simulink library "RxTxFixedPointLibrary"  (R2018a)
settings: Solver=VariableStepAuto  StartTime=0.0  StopTime=10.0  RelTol=1e-3
values from neighbouring files (symbols this model uses):
  AGCBarkerSymbols = 160 + 28    (= 188)    [modelSettings.m]
  coeff = rcosdesign(beta, span, sps, 'sqrt') * filterGain    [modelSettings.m]
  crcDecodeLag = length(crc32Poly) - 1 + 2    [modelSettings.m]
  CRCGeneratorLag = 34    [modelSettings.m]
  EQTrainingSymbols = 250    [modelSettings.m]
  K1 = fi(K1, 0)    [modelSettings.m]
  K2 = fi(K2, 0)    [modelSettings.m]
  numHeaderBits = 16    [modelSettings.m]
  numTrainingSamples = 250    [modelSettings.m]
  pLen = uint16(length(PreambleBarkersBits))    [modelSettings.m]
  RadioSampleRate = 1e6    (= 1000000)    [modelSettings.m]
  samplesPerSymbol = 4    [modelSettings.m]
  VibertiTracebackLength = 34 + 0    (= 34)    [modelSettings.m]
  xPreambleSeq = hPSKModTrain(seq)    [modelSettings.m]
undefined symbols (not defined in the file or in its folder): j
libraries: simulink x25, dsphdlfiltering x20, hdlsllib x10, commseqgen3 x4, commdigbbndpm3 x3, commcrc2 x2, commcnvcod2 x2, dspsigops x2, dspstat3 x1, commfilt2 x1
(part 3 of 3)

== matlab function RxTxFixedPointLibrary/Receiver_HDL/Viterbi Decode/Buffer/DEBUG: Vitberi Check/MATLAB Function2 ==
  data: bits input; enable input; reset input; crc input
function fcn(bits, enable, reset, crc)
 
persistent buffer index crcEnc crcDec txData

trellis = poly2trellis(7,[171 133]);
tbl = 34;

if isempty(buffer)
    buffer = false(4000,1);
    index = uint16(1);
    ply = 'z^32 + z^26 + z^23 + z^22 + z^16 + z^12 + z^11 + z^10 + z^8 + z^7 + z^5 + z^4 + z^2 + z + 1';
    crcEnc = comm.CRCGenerator('Polynomial',ply);
    crcDec = comm.CRCDetector ('Polynomial',ply);
    rate = 1/2;
    txData = repmat(logical([0;1]), 8*200*log2(4)*rate/2, 1); % Repeating [0 1]
end

if enable
    if reset
       index = uint16(1); 
    end
    
    buffer(index:index+1) = bits;
    index = index + uint16(2);
    if crc%index>3480
        % Generate true data
        crctx = crcEnc(txData);
        dataHardtx = convenc(crctx,trellis);
        % Check
        crcrx = vitdec(buffer(1:3264+tbl*2),trellis,tbl,'cont','hard');
        [rxData,e2] = crcDec(crcrx(tbl+1:tbl+1632));
        % Double check
        crcrx2 = vitdec([dataHardtx;false(tbl*2,1)],trellis,tbl,'cont','hard');
        [rxData2,e2] = crcDec(crcrx2(tbl+1:tbl+1632));
        %[dataHardtx buffer(1:3264)]
        disp(e2);
    end
    if index>4000
        index = uint16(1);
    end
end

== matlab function RxTxFixedPointLibrary/Transmitter_HDL/Packet Generation/Payload/MATLAB Function ==
  data: enable input; reset output; mode output
function [reset,mode] = fcn(enable)

persistent counter

if isempty(counter)
   counter = uint8(0);
end

if enable
    counter = uint8(34*2); % tracebacklength*2
    mode = uint8(1);
    reset = true;
elseif counter>uint8(0)
    counter = counter - 1;
    mode = uint8(1);
    reset = false;
else
    mode = uint8(0);
    reset = false;
end

== matlab function RxTxFixedPointLibrary/Receiver_HDL/Frame Recover/Gardner Timing Recovery/TED Lock Detector/MATLAB Function ==
  data: u input; y output
function y = abs(u)

y = fi(u,0,16,15);

== matlab function RxTxFixedPointLibrary/Receiver_HDL/CRC Check and DMA Pack/CRC Check ES/DEBUG: Check CRC Result ==
  data: bits input; start input; done input; valid input; err input
function fcn(bits, start, done, valid, err)

persistent buffer

if isempty(buffer)
    buffer = fi(false(1032,1),0,1,0);
end

buffer = [buffer(2:end);bits];

if done && valid
    if err
        fprintf('CRC Error (HDL CRC)\n');
    else
        fprintf('CRC Passed (HDL CRC)\n');
    end
end
if err % Flag if any error every occurs, if it occurs alone it means given crc is not long enough
    fprintf('CRC Error Type 2 (HDL CRC)\n');
end

== matlab function RxTxFixedPointLibrary/Receiver_HDL/CRC Check and DMA Pack/CRC Check ES/DEBUG: CRC Input ==
  data: u input; enable input; endFlag input; startFlag input
function fcn(u, enable,endFlag,startFlag)

persistent buffer crc count
%persistent crcd

if isempty(buffer)
   buffer = false(3000,1); 
    crc = comm.CRCDetector('Polynomial','z^32 + z^26 + z^23 + z^22 + z^16 + z^12 + z^11 + z^10 + z^8 + z^7 + z^5 + z^4 + z^2 + z + 1');
%    crcd = comm.CRCGenerator('Polynomial','z^32 + z^26 + z^23 + z^22 + z^16 + z^12 + z^11 + z^10 + z^8 + z^7 + z^5 + z^4 + z^2 + z + 1');
    count = 1;
end

if enable
    %buffer = [buffer(2:end);u];
    if startFlag
        count = 1;
    elseif count>3000-1
        count = 1;
    else
        count = count + 1;
    end
    buffer(count) = u;
    
    if endFlag
%        disp(count)
        payloadBytes = 8*25;
        k = buffer(1:payloadBytes*8+32);%1632
%         cc = k(end-31:end);
%         front = k(1:64);
%         mid = k(  (65:64+(payloadBytes-2*8)*8) );
%         back = k(end-31-64:end-32);
%         p = crcd(buffer(1:payloadBytes*8));
        [~,e] = crc(k);
        if e
            fprintf('Pre CRC Check Error (at %d)\n',int32(count));
        else
            fprintf('Pre CRC Check Pass (at %d)\n',int32(count));
        end
    end
    
end

== matlab function RxTxFixedPointLibrary/Transmitter_HDL/Packet Generation/Payload/Subsystem/MATLAB Function3 ==
  data: start input; enable output; done input
function enable = latch(start,done)

persistent state

if isempty(state)
   state = false; 
end

if start
    enable = true;
    state = true;
elseif done
    enable = true;
    state = false;
else
    enable = state;
end

== matlab function RxTxFixedPointLibrary/Receiver_HDL/Frame Recover/Equalization and Demodulation/2 Bit Descrambler/MATLAB Function ==
  data: bits input; bufferA output; reset input; bufferB output
function [bufferA, bufferB] = BufferSelect(bits,reset)

persistent buffer

% Constants
initBuffer = logical([0 1 0 0 0 1 0]);

% Async
if isempty(buffer)
    buffer = initBuffer;
end

% Reset/Sync
if reset
    bufferA = initBuffer;
    bufferB = [bits(1),initBuffer(1:end-1)];
    buffer = [bits(2),bits(1),initBuffer(1:end-2)];
else
    bufferA = buffer;
    bufferB = [bits(1),buffer(1:end-1)];
    buffer = [bits(2),bits(1),buffer(1:end-2)];    
end

== matlab function RxTxFixedPointLibrary/Receiver_HDL/CRC Check and DMA Pack/DMA Interface/Bit Packer ==
  data: bitIn input; byteOut output; startIn input; endIn input; err input; validIn input; validOut output; startOut output
function [byteOut,validOut,startOut] = BitPacker(bitIn, startIn, endIn, err, validIn)

% This block will pack bits into bytes with start boundaries


% Constants
bits2Pack = uint8(64); % byteReg must contain this many bits
zero64 = fi(0,0,64,0);
% NOTE: Frames but be a multiple of bits2Pack or bits will be trimmed from
% end

persistent byteReg byteIndx setStartFlag

if isempty(byteIndx)
    byteReg  = fi(0,0,64,0);
    byteIndx = uint8(1);
    setStartFlag = false;
end

if validIn
    if startIn % Reset
        byteReg = bitset(zero64,1,bitIn);
        byteIndx = uint8(2);
        validOut = false;
        setStartFlag = true;
        startOut = false;
    else
        byteReg = bitset(byteReg,byteIndx,bitIn);
        if byteIndx >= bits2Pack
            byteIndx = uint8(1);
            validOut = true;
            startOut = setStartFlag;
            setStartFlag = false;
        else
            byteIndx = byteIndx + uint8(1);
            validOut = false;
            startOut = false;
        end
    end
elseif endIn % Append error bit to last byte
    byteReg = fi(err,0,64,0);
    validOut = true;
    startOut = false;
else
    validOut = false;
    startOut = false;
end

byteOut = byteReg;

== matlab function RxTxFixedPointLibrary/Receiver_HDL/Frame Recover/Enable Equalizer and Packet Decode (Latch) ==
  data: start input; enable output; validIn input
function enable = Counter(start,validIn)

persistent count maxCount lastEOF

if isempty(count)
    count = uint32(0);
    maxCount = uint32(2^16); % Largest possible packet length
    lastEOF = false;
end

eof = false;

if validIn
    % Got a barker preamble start allowing data into equalizer
    if start
        count = maxCount;
    end
    
    % Check on change from true to false
    if lastEOF && ~eof
        %     fprintf('Frame end reached\n');
        count = uint32(0);
    end
    lastEOF = eof;
    
    % Past end of max frame size
    if count>0
        count = count - uint32(1);
    end
    
    % Enable downstream
    enable = count>uint32(0);
else
    enable = false;
end

== matlab function RxTxFixedPointLibrary/Receiver_HDL/Frame Recover/Manage Error Signals/Subsystem/DEBUG: Header ==
  data: status input; h1 input; h2 input
function HeaderDebug(status,h1,h2)

if status==uint8(2)
    fprintf('Header Check failed (possible false detection)\n');
    fprintf('sum1: %d\n',int32(h1));
    fprintf('sum2: %d\n',int32(h2));
elseif status==uint8(1)
    fprintf('Header Found | Packet is %d bits long\n',int32(h1));
end

== matlab function RxTxFixedPointLibrary/Receiver_HDL/Frame Recover/Equalization and Demodulation/DFE/Equalizer ==
  data: trigger input; eqOut output; data input; trainingSymbol input
function eqOut  = dfe(trigger,data,trainingSymbol)

persistent inputBuffer decisionBuffer forwardTaps backwardTaps processedSamples


%% Constants
WL = uint8(16); FL = uint8(14);
F = fimath('SumMode','SpecifyPrecision','SumWordLength',WL,...
    'SumFractionLength',FL);
% Initial delay guess
channelDelay = uint8(0);
% Equalizer settings
mu = fi(0.05,0,10,12);
nFTaps = uint8(11);
nBTaps = uint8(3);
numTrainingSymbols = uint16(250);
resetTaps = fi([complex(zeros(nFTaps-1,1));1],1,WL,FL,F);

%% Async
if isempty(inputBuffer)
    % Set Precisions
    inputBuffer = fi(complex(zeros(nFTaps,1)),1,WL,FL,F);
    decisionBuffer = fi(complex(zeros(nBTaps,1)),1,WL,FL,F);
    forwardTaps = fi(complex(zeros(nFTaps,1)),1,WL,FL,F);
    backwardTaps = fi(complex(zeros(nBTaps,1)),1,WL,FL,F);
    processedSamples = numTrainingSymbols + uint16(1); % Force to DD mode to start
end

%% Reset
if trigger
    processedSamples = uint16(0);
    % Reset taps
    %forwardTaps = fi(complex(zeros(nFTaps,1)),1,WL,FL,F);
    %forwardTaps(nFTaps-channelDelay) = fi(1,1,WL,FL); % Favor specific delay (causes equalizer to converge faster)
    forwardTaps = resetTaps;
    backwardTaps = fi(complex(zeros(nBTaps,1)),1,WL,FL,F);
    % Default output
    eqOut = fi(0,1,WL,FL,F);
else
    %% Equalizer
    % Add data to buffer
    inputBuffer = [inputBuffer(2:end);data];
    
    % Apply equalizer
    eqOut = forwardTaps'*inputBuffer - backwardTaps'*decisionBuffer;
    
    % Determine error
    if (processedSamples<numTrainingSymbols) && (processedSamples>=channelDelay)
        processedSamples = processedSamples + 1;
        d = trainingSymbol;
    else % Decision directed
        % Find closest symbol
        r = real(eqOut)>0; i = imag(eqOut)>0;
        if r
            if i
                d = fi(0.7071 + 0.7071i,1,WL,FL);
            else
                d = fi(0.7071 - 0.7071i,1,WL,FL);
            end
        else
            if i
                d = fi(-0.7071 + 0.7071i,1,WL,FL);
            else
                d = fi(-0.7071 - 0.7071i,1,WL,FL);
            end
        end
    end
    ec = conj(d - eqOut);
    
    % Update taps
    forwardTaps = forwardTaps + mu*ec*inputBuffer;
    backwardTaps = backwardTaps - mu*ec*decisionBuffer;
    
    % Update decision buffer
    db = fi(d,1,WL,FL,F);
    decisionBuffer = [db; decisionBuffer(1:end-1)];
    
end



end

== matlab function RxTxFixedPointLibrary/Receiver_HDL/Frame Recover/Equalization and Demodulation/Header Controller ==
  data: enableDownstream output; headerStart input; packetLenBitsOut output; data input; resetViterbi output; crcStart output; status output; s1 output; s2 output
function [enableDownstream,packetLenBitsOut,resetViterbi,crcStart,status,s1,s2] = EvalHeader(headerStart, data)

persistent counter sum1 sum2 packetLenBits lastMode savedPacketLenBits

% The header contains 16 bits, but each bit is duplicated to make checking
% easier
%
% Note this block works on symbols (2bits) but 1 symbol -> 1 decoded bit
%
% PacketLength = (Data+CRC+40(TB)+68)/CodeRate
%
% NOTE TAIL BITS HERE ARE REALLY USED TO DEAL WITH VITERBI LAG SO:
% TailBitsWithLagPadding > TracebackLength

%% Constants
numHeaderBits = uint8(16); % Header is this many bits
powersOfTwo = uint32([1 2 4 8 16 32 64 128 256 512 1024 2048 4096 8192 16384 32768]);
CodeRateINV = uint32(2);%1/CodeRate;
TailBitsWithLagPadding = uint32(uint32(40)+34*2+1); % was +1
% Flag when CRC porition of packet starts relative to header
crcSignalStartLocation = uint32((TailBitsWithLagPadding)*CodeRateINV); % Must be even

% Async
if isempty(counter)
    packetLenBits = uint32(0);
    sum1 = uint32(0);
    sum2 = uint32(0);
    counter = uint8(numHeaderBits);
    lastMode = uint8(3);
    savedPacketLenBits = uint16(0);
end


%% Sync
% Got a header now enable certain mode
if headerStart
    mode = uint8(0);
else
    mode = lastMode;
end

switch mode
    %% Reset on preamble flag and setup for header processing
    case uint8(0)
        crcStart = false;
        resetViterbi = false;
        enableDownstream = false;
        sum1 = uint32(0);
        sum2 = uint32(0);
        counter = uint8(1);
        lastMode = uint8(1); % Go to next state
        packetLenBitsOut = uint16(0);
        status = uint8(0); s1 = uint32(0); s2 = uint32(0);
        
    %% Process header
    case 1 
        crcStart = false;
        enableDownstream = false;
        
        % Convert header bits (bit by bit)
        if data(1)
            sum1 = sum1 + powersOfTwo(counter);
        end
        if data(2)
            sum2 = sum2 + powersOfTwo(counter);
        end
        counter = counter + uint8(1);
        
        if counter>numHeaderBits
            % Check header
            if sum1~=sum2 % Fail
                packetLenBits = uint32(0);
                lastMode = uint8(3);
                resetViterbi = false;
                packetLenBitsOut = uint16(0);
                savedPacketLenBits = uint16(0);
                status = uint8(2); s1 = sum1; s2 = sum2;
            else % Pass
                % Saved header info and trigger downstream
                packetLenBits = uint32(sum1);
                lastMode = uint8(2);
                resetViterbi = true;
                packetLenBitsOut = uint16(sum1-crcSignalStartLocation);
                savedPacketLenBits = uint16(sum1-crcSignalStartLocation);
                status = uint8(1); s1 = sum1; s2 = sum2;
            end
        else
            status = uint8(0); s1 = uint32(0); s2 = uint32(0);
            packetLenBitsOut = uint16(0);
            resetViterbi = false;
        end
        
    %% Decrement sample counter
    case 2 
        status = uint8(0); s1 = uint32(0); s2 = uint32(0);
        resetViterbi = false;
        crcStart = (packetLenBits==crcSignalStartLocation);
        if packetLenBits>uint32(0)
            enableDownstream = true;
            packetLenBits = packetLenBits - uint32(2); % We get 2 bits each call
            packetLenBitsOut = savedPacketLenBits;
        else
            enableDownstream = false;
            lastMode = uint8(3);
            packetLenBitsOut = uint16(0); %Reset
            savedPacketLenBits = uint16(0);%Reset
        end
            
    %% Not processing anything
    otherwise % mode>2
        status = uint8(0); s1 = uint32(0); s2 = uint32(0);
        crcStart = false;
        resetViterbi = false;
        enableDownstream = false;
        packetLenBitsOut = uint16(0);
end

== matlab function RxTxFixedPointLibrary/Receiver_HDL/Frame Recover/Frequency Recovery/PED ==
  data: In input; e output
function e  = PED(In)

OP2 = real(In);
OP1 = imag(In);

Real = OP2;
Imag = OP1;

if (bitget(Real,16)==true) % real component is negative
    OP1 = fi(-Imag,1,16,13);
end
if (bitget(Imag,16)==true) % imaginary component is negative
    OP2 = fi(-Real,1,16,13);
end

e= fi(OP1-OP2,1,16,10);

%e = sign(real(In)).*imag(In) - sign(imag(In)).*real(In);

== matlab function RxTxFixedPointLibrary/Transmitter_HDL/DMA Interface/DMA Control ==
  data: byteIn input; bitOut output; validIn input; validOut output; startOut output; payloadLength output; readyForInput output; EOF input
function [bitOut,validOut,startOut,payloadLength,readyForInput] = DMA_Control(byteIn,validIn,EOF)

% This block converts the byte input pipeline into bits and extract the
% length the packet into its own signal

persistent wordBuffer bitCounter payloadLenBuff mode inputByteCounter

bitsInInput = uint8(64);
bytesInInput = uint16(8);

if isempty(wordBuffer)
    wordBuffer = fi(0,0,64,0); % Must match number of bits defined by bitsInInput
    bitCounter = uint8(0);
    payloadLenBuff = uint16(0);
    mode = uint8(0);
    inputByteCounter = uint16(0);
end

%% Payload length setup
% Capture first payload length byte(s)
if validIn && (mode == uint8(0))
    mode = uint8(2);
    payloadLenBuff = uint16(byteIn);
    % Set outputs
    bitOut = false;
    validOut = false;
    startOut = true;
    payloadLength = uint16(0);
    readyForInput = true;
    % Reset counters
    inputByteCounter = bytesInInput;% Reset
    bitCounter = uint8(1);% Reset
    
%% Payload output
elseif (bitCounter > uint8(0))  && (mode==uint8(2))
    % Set outputs
    if bitCounter==uint8(1)
        bitOut = bitget(byteIn,1)>0;
        wordBuffer = byteIn; % Save byte
    else
        bitOut = bitget(wordBuffer,bitCounter)>0;
    end
    startOut = false;
    payloadLength = uint16(payloadLenBuff);
    validOut = true;
    % Set flag to DMA and next mode
    if bitCounter >= uint8(bitsInInput)
        bitCounter = uint8(1); % Reset
        % If we've processed all the bytes we need to wait for downstream
        % to be done
        if inputByteCounter<payloadLenBuff
            readyForInput = true; % Tell them we need next byte
            % Bytes processed
            inputByteCounter = inputByteCounter + bytesInInput;    
        else
            readyForInput = false; % Hold DMA off for now, next call will go to EOF
            mode = uint8(3);
        end
    else
        bitCounter = bitCounter+uint8(1);
        readyForInput = false;
    end
    
% Waiting for EOF from packet generation
elseif (mode==uint8(3))
    bitOut = false;
    validOut = true; % Keep downstream processing going
    startOut = false;
    payloadLength = uint16(payloadLenBuff);
    if EOF % Done with frame now ask for more data
        readyForInput = true;
        mode = uint8(0);% Reset
    else
        readyForInput = false;
    end
    
else % not-valid and need another byte
    bitOut = false;
    if mode == uint8(0)
        validOut = true; % Let LFSR Run
    else
        validOut = false;
    end
    startOut = false;
    payloadLength = uint16(0);
    readyForInput = true;
end

== matlab function RxTxFixedPointLibrary/Transmitter_HDL/Packet Generation/Payload/Enable Latch/MATLAB Function ==
  data: startpacket input; outEnable output; endpacket input
function outEnable = fcn(startpacket,endpacket)

persistent enable

if isempty(enable)
    enable = false;
end

% Latch
if startpacket
    enable = true;
    outEnable = true;
elseif endpacket
    enable = false;
    outEnable = true;
else
    outEnable = enable;
end

== matlab function RxTxFixedPointLibrary/Transmitter_HDL/Packet Generation/Payload/HDL Scrambler 2 bits/Buffer Manage ==
  data: bit1 input; bit2 input; outBuffer output; reset input
function outBuffer = fcn(bit1, bit2, reset)
%#codegen

init_buffer = logical([0 1 0 0 0 1 0]);

persistent buffer

if isempty(buffer)
    buffer = init_buffer;
end

if reset
    outBuffer = init_buffer;
    buffer = init_buffer;
    %outBuffer = [init_buffer(3:end),bit1,bit2];
    %buffer = [buffer(3:end),bit1,bit2];    
else
    outBuffer = [bit2,bit1,buffer(1:end-2)];
    buffer = [bit2,bit1,buffer(1:end-2)];
end

== matlab function RxTxFixedPointLibrary/Transmitter_HDL/Packet Generation/Tx Controller ==
  data: modeOut output; headerData output; data output; payloadBit input; payloadSize input; count input; start input; dataStart output; dataEnd output; preambleReset output
function [modeOut, headerData, data, dataStart, dataEnd, preambleReset] = fcn(payloadBit,payloadSize,count, start)

% When we get a start flag buffers are reset and the next cycle with start
% in mode 0

% Reset: New payload size is passed at an int16
% 


persistent  headerBits numPayloadBits mode

numHeaderBits = uint32(16);
AGCBarkerSymbols = 160+28;
EQTrainingSymbols = 250; % 2 bits per symbol => 250 symbols
preambleBits = uint32(EQTrainingSymbols+AGCBarkerSymbols-0);
CRCLength = 32;
CRCGeneratorLag = CRCLength+2+0; % additional 1 is from reset of encoder
CodeRate = 2;
lagBits = 40+68;
viterbiTraceback = uint32(34*2);

% Async/Init
if isempty(numPayloadBits)
    % Sizes of frame sections
    numPayloadBits = uint32(0); 
    %headerBits = zeros(1,numHeaderBits)>0;
    headerBits = uint16(0);
    mode = uint8(4);
end

% Synchronous
switch mode
    case uint8(0) % Reset
        % Move to next mode on next input/clock
        mode = uint8(1);
        % Convert payloadSize to bits
        numPayloadBits = uint32(bitshift(payloadSize,3)+CRCLength);
        %headerBits = logical(bitget(CodeRate*(payloadSize+CRCLength),1:numHeaderBits));
        headerBits = uint16(bitshift((bitshift(payloadSize,3)+CRCLength+lagBits),1));        
        % Set outputs
        modeOut = uint8(4);
        headerData = false;
        data = false; % Not used downstream
        dataStart = false;
        dataEnd = false;
        preambleReset = true;
    case uint8(1) % Preamble
        % Set Next Mode
        if count>=(preambleBits)
            preambleReset = false;
            mode = uint8(2);
        elseif count==uint32(1)
            preambleReset = false;
            mode = uint8(1);
        else
            preambleReset = false;
            mode = uint8(1);
        end
        % Set outputs
        modeOut = uint8(1);
        headerData = false;
        % Start outputing data early to compensate for CRC lag
        if count>=(preambleBits+numHeaderBits-CRCGeneratorLag)
           data = payloadBit;
           % Set flag on first payload bit
           dataStart = count == (preambleBits+numHeaderBits-CRCGeneratorLag);
        else
           data = false;         
           dataStart = false;
        end
        dataEnd = false;
    case uint8(2) % Header bits
        % Set Next Mode
        if count>=(preambleBits+numHeaderBits)
            mode = uint8(3);
        else
            mode = uint8(2);
        end
        % Set outputs
        modeOut = uint8(2);
        %headerData = headerBits(count-preambleBits);
        headerData = bitget(headerBits,count-preambleBits)>0;
        data = payloadBit;
        dataStart = false;
        dataEnd = false;
        preambleReset = false;
    case uint8(3) % Payload bits and CRC
        % Set Next Mode
        if count>=(preambleBits+numHeaderBits+numPayloadBits+viterbiTraceback)%+CRCGeneratorLag)
            % Will coencide with last CRC Bit (NOT TRUE ANYMORE WILL BE ON
            % LAST TRACEBACK PADDING BIT)
            mode = uint8(4);
        else
            mode = uint8(3);
        end
        % Set outputs
        modeOut = uint8(3);        
        headerData = false;
        data = payloadBit;
        % Set flag on last payload bit
        dataStart = false;
        dataEnd =   ( count==(preambleBits+numHeaderBits+numPayloadBits-CRCLength-CRCGeneratorLag-1) );
        preambleReset = false;
    otherwise %case uint8(4) % Waiting for data
        % Chilling for new start
        if start
           mode = uint8(0); 
        else
           mode = uint8(4);
        end
        % Set outputs
        modeOut = uint8(4);
        headerData = false;
        data = false; % Not used downstream
        dataStart = false;
        dataEnd = false;
        preambleReset = false;
end

== matlab function RxTxFixedPointLibrary/Receiver_HDL/Viterbi Decode/Buffer/MATLAB Function ==
  data: valid input; enable output; start input; crcEnd input
function enable = latch(valid,start,crcEnd)

persistent state

if isempty(state)
    state = false;
end

if start
    enable = true && valid;
    state = true;
elseif crcEnd
    enable = true && valid;
    state = false;
else 
    enable = state && valid;
end
